simulink model "ex_anti_windup_op_PID"  (R2024a)
settings: Solver=VariableStepAuto  StartTime=0.0  StopTime=100  MaxStep=0.01  RelTol=1e-3
StopFcn:
  | figure(1);
  | 
  | subplot(211);
  | plot(r.time,r.data,y.time,y.data);
  | ylabel('r, y');
  | xlabel('Temps (s)');
  | 
  | subplot(212);
  | plot(u.time,u.data);
  | ylabel('u');
  | xlabel('Temps (s)');
  | 
  | figure(2);
  | 
  | subplot(211);
  | plot(e.time,e.data);
  | ylabel('e');
  | xlabel('Temps (s)');
  | 
  | subplot(212);
  | plot(ef.time,ef.data);
  | ylabel('ef');
  | xlabel('Temps (s)');
settings Model: Creator=eric  LastModifiedBy=sabri
settings SolverCC: AlgebraicLoopSolver=TrustRegion
settings DataIOCC: SaveTime=off  ReturnWorkspaceOutputs=off
settings DebuggingCC: UnconnectedInputMsg=warning  UnconnectedOutputMsg=warning  UnconnectedLineMsg=warning
settings ModelReferenceCC: EnableRefExpFcnMdlSchedulingChecks=on
settings RTWCC: GPUComputeCapability=3.5

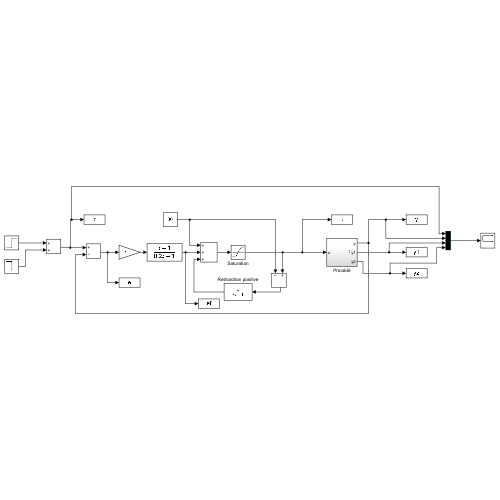
[thumbnail: Simulink's stored preview of the top-level diagram]
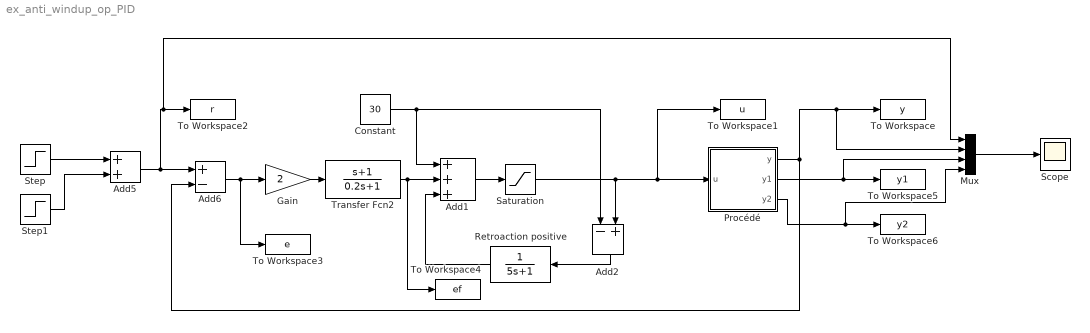
== system ex_anti_windup_op_PID ==
  Add1 : Sum  Inputs=+++
  Add2 : Sum  Inputs=-+
  Add5 : Sum
  Add6 : Sum  Inputs=+-
  Constant : Constant  Value=30
  Gain : Gain  Gain=2
  Mux : Mux
  Procédé : Subsystem
  Retroaction positive : TransferFcn  Denominator=[5 1]
  Saturation : Saturate  UpperLimit=40  LowerLimit=0
  Scope : Scope
  Step : Step  Time=10  Before=22  After=32  SampleTime=0
  Step1 : Step  Time=60  After=-5  SampleTime=0
  To Workspace : ToWorkspace  VariableName=y  SaveFormat=Timeseries  SampleTime=-1
  To Workspace1 : ToWorkspace  VariableName=u  SaveFormat=Timeseries  SampleTime=-1
  To Workspace2 : ToWorkspace  VariableName=r  SaveFormat=Timeseries  SampleTime=-1
  To Workspace3 : ToWorkspace  VariableName=e  SaveFormat=Timeseries  SampleTime=-1
  To Workspace4 : ToWorkspace  VariableName=ef  SaveFormat=Timeseries  SampleTime=-1
  To Workspace5 : ToWorkspace  VariableName=y1  SaveFormat=Timeseries  SampleTime=-1
  To Workspace6 : ToWorkspace  VariableName=y2  SaveFormat=Timeseries  SampleTime=-1
  Transfer Fcn2 : TransferFcn  Numerator=[1 1]  Denominator=[0.2 1]
  wires:
  Step/1 -> Add5/1
  Add6/1 -> To Workspace3/1, Gain/1
  Add1/1 -> Saturation/1
  Saturation/1 -> To Workspace1/1, Procédé/1(u), Add2/2
  Add2/1 -> Retroaction positive/1
  Constant/1 -> Add2/1, Add1/1
  Retroaction positive/1 -> Add1/3
  Step1/1 -> Add5/2
  Add5/1 -> Mux/1, To Workspace2/1, Add6/1
  Procédé/1(y) -> Add6/2, Mux/2, To Workspace/1
  Transfer Fcn2/1 -> To Workspace4/1, Add1/2
  Gain/1 -> Transfer Fcn2/1
  Procédé/2(y1) -> Mux/3, To Workspace5/1
  Procédé/3(y2) -> Mux/4, To Workspace6/1
  Mux/1 -> Scope/1

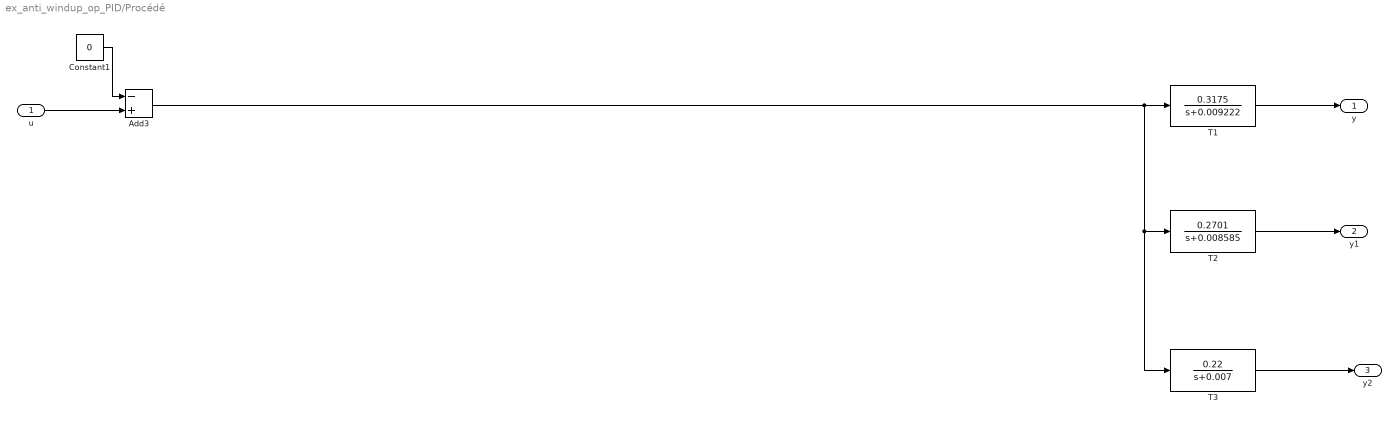
== system ex_anti_windup_op_PID/Procédé ==
  u : Inport
  Add3 : Sum  Inputs=-+
  Constant1 : Constant  Value=0
  T1 : TransferFcn  Numerator=[0.3175]  Denominator=[1 0.009222]
  T2 : TransferFcn  Numerator=0.2701  Denominator=[1 0.008585]
  T3 : TransferFcn  Numerator=[0.22]  Denominator=[1 0.007]
  y : Outport
  y1 : Outport  Port=2
  y2 : Outport  Port=3
  wires:
  u/1 -> Add3/2
  T1/1 -> y/1
  Constant1/1 -> Add3/1
  T2/1 -> y1/1
  T3/1 -> y2/1
  Add3/1 -> T3/1, T2/1, T1/1
